simulink model "nms_3Dmodel_forward_no_rbld"  (R2017b)
settings: Solver=VariableStepAuto  StartTime=0.0  StopTime=t_end  FixedStep=1e-4  MinStep=1e-9  RelTol=1e-2  AbsTol=1e-3  EnableMultiTasking=on
InitFcn:
  | runScripts;
values from neighbouring files (symbols this model uses):
  ankle_height = 0.08    [nms_MechInit.m]
  ankleIMP = param(91+length(paramIC_opt):93+length(paramIC_opt))    [runScripts.m]
  c = 0.05    [IID_nms_MechInit.m]    (also in nms_MechInit.m)
  c_jointstop = 0.3 / (pi/180)    (= 17.1887338539)    [IID_nms_MechInit.m]    (also in nms_MechInit.m)
  CPG_On = 0    [setCPGPar.m]    (also in setCPGPar_inv.m = 1)
  CtrlPar_FP = [alpha0 alpha_cd alpha_cv]    [setCtrlPar.m]
  CtrlPar_FP_R = [R_hipR0 R_hipR_cd R_hipR_cv]    [setCtrlPar.m]
  CtrlPar_LL = l_clr    [setCtrlPar.m]
  CtrlPar_Side = [beta_cd  beta_cv]    [setCtrlPar.m]
  CtrlPar_St = [StPreStim St_M1 St_M2 St_M3 St_M4 St_M5 St_M11]    [setCtrlPar.m]
  CtrlPar_St_R = [R_StPreStim R_St_M1 R_St_M3 R_St_M4]    [setCtrlPar.m]
  CtrlPar_Sw = [SwPreStim SwPhasePari SwPhaseParii SwCtrlPar_H SwCtrlPar_A      SwCtrlPar_Ki SwCtrlPar_Kii SwCtrlPar_Kiii SwCtrlPar_StP]    [setCtrlPar.m]
  CtrlPar_Sw_R = [R_SwPreStim R_Sw_M6]    [setCtrlPar.m]
  CtrlPar_theta0 = parBlCtrl(1)      *1*pi/180    [setCtrlPar.m]
  CtrlPar_Tr = [Tr_St_sup Tr_Sw]    [setCtrlPar.m]
  CtrlPar_Tr_R = [R_Tr_St_sup R_Tr_Sw]    [setCtrlPar.m]
  D12_F = 0.16    [IID_nms_MechInit.m]    (also in nms_MechInit.m)
  D12_S = L_S    (= 0.5)    [IID_nms_MechInit.m]    (also in nms_MechInit.m = 0.46)
  D12_T = L_T    (= 0.5)    [IID_nms_MechInit.m]    (also in nms_MechInit.m = 0.46)
  D12z_T = 0.1* scalorFactor    (= 0.1)    [nms_MechInit.m]
  D13_F = 0.20    (= 0.2)    [IID_nms_MechInit.m]    (also in nms_MechInit.m)
  D1G_F = 0.14    [IID_nms_MechInit.m]    (also in nms_MechInit.m)
  D1G_HAT = 0.35    [IID_nms_MechInit.m]    (also in nms_MechInit.m)
  D1G_S = 0.3    [IID_nms_MechInit.m]    (also in nms_MechInit.m = 0.28)
  D1G_T = 0.3    [IID_nms_MechInit.m]    (also in nms_MechInit.m = 0.28)
  D1Gy_F = ankle_height*D1G_F/D12_F    (= 0.07)    [nms_MechInit.m]
  d_fBall = 0.1    [nms_MechInit.m]
  d_fHeel = 0.05    [nms_MechInit.m]
  DeltaThRef = 5e-3    (= 0.005)    [IID_nms_MechInit.m]    (also in nms_MechInit.m)
  Dist_LM23_PH = 0    [setDistPar.m]
  Dist_LM34_PH = 0    [setDistPar.m]
  Dist_On = 1    [IID_setDistPar.m]    (also in setDistPar.m)
  Dist_PDur = 0.15    [IID_setDistPar.m]    (also in setDistPar.m)
  Dist_RM23_PH = 0    [setDistPar.m]
  Dist_RM34_PH = 0    [setDistPar.m]
  Dist_StartTime = 15    [IID_setDistPar.m]    (also in setDistPar.m)
  Dist_xyzHAT_front_PH = 0    [setDistPar.m]
  Dist_xyzHAT_sag_PH = 0    [IID_setDistPar.m]    (also in setDistPar.m)
  Dist_xyzLAnkle_PH = 0    [setDistPar.m]
  Dist_xyzRAnkle_PH = 0    [setDistPar.m]
  eref = 0.04    [IID_nms_MechInit.m]    (also in nms_MechInit.m)
  FmaxBFSH = 350    [nms_MechInit.m]
  FmaxGAS = 1500    [IID_nms_MechInit.m]    (also in nms_MechInit.m)
  FmaxGLU = 1500    [IID_nms_MechInit.m]    (also in nms_MechInit.m)
  FmaxHAB = 3000    [nms_MechInit.m]
  FmaxHAD = 4500    [nms_MechInit.m]
  FmaxHAM = 3000    [IID_nms_MechInit.m]    (also in nms_MechInit.m)
  FmaxHFL = 2000    [IID_nms_MechInit.m]    (also in nms_MechInit.m)
  FmaxRF = 1200    [nms_MechInit.m]
  FmaxSOL = 4000    [IID_nms_MechInit.m]    (also in nms_MechInit.m)
  FmaxTA = 800    [IID_nms_MechInit.m]    (also in nms_MechInit.m)
  FmaxVAS = 6000    [IID_nms_MechInit.m]    (also in nms_MechInit.m)
  In_F = 0.005    [IID_nms_MechInit.m]    (also in nms_MechInit.m)
  In_HAT = 3    [IID_nms_MechInit.m]    (also in nms_MechInit.m = 2.5)
  In_S = 0.05    [IID_nms_MechInit.m]    (also in nms_MechInit.m)
  In_T = 0.15    [IID_nms_MechInit.m]    (also in nms_MechInit.m)
  init_a_tgt = 70*pi/180    (= 1.2217304764)    [setInitPar.m]
  init_a_tgtR = 90*pi/180    (= 1.57079632679)    [setInitPar.m]
  Inx_F = 0.0007    [nms_MechInit.m]
  Inx_HAT = 1.0    (= 1)    [nms_MechInit.m]
  Inx_S = 0.003    [nms_MechInit.m]
  Inx_T = 0.03    [nms_MechInit.m]
  Iny_F = 0.005    [nms_MechInit.m]
  Iny_HAT = 4.0    (= 4)    [nms_MechInit.m]
  Iny_S = 0.05    [nms_MechInit.m]
  Iny_T = 0.15    [nms_MechInit.m]
  K = 5    [IID_nms_MechInit.m]    (also in nms_MechInit.m)
  k_gn = k_gn/2    (= 39240)    [nms_MechInit.m]
  k_gt = k_gt/2    (= 3924)    [nms_MechInit.m]
  k_pressure = m_HAT * 9.81 / DeltaThRef    (= 104967)    [IID_nms_MechInit.m]    (also in nms_MechInit.m)
  leg_l = [D12_T D12_S]    [nms_MechInit.m]
  LongDelay = 0.020    (= 0.02)    [IID_setCtrlPar.m]    (also in nms_MechInit.m = 0.01)
  LongLoopDelay = 0.030    (= 0.03)    [nms_MechInit.m]
  loptBFSH = 0.12    [nms_MechInit.m]
  loptGAS = 0.05    [IID_nms_MechInit.m]    (also in nms_MechInit.m)
  loptGLU = 0.11    [IID_nms_MechInit.m]    (also in nms_MechInit.m)
  loptHAB = 0.09    [nms_MechInit.m]
  loptHAD = 0.10    (= 0.1)    [nms_MechInit.m]
  loptHAM = 0.10    (= 0.1)    [IID_nms_MechInit.m]    (also in nms_MechInit.m)
  loptHFL = 0.11    [IID_nms_MechInit.m]    (also in nms_MechInit.m)
  loptRF = 0.08    [nms_MechInit.m]
  loptSOL = 0.04    [IID_nms_MechInit.m]    (also in nms_MechInit.m)
  loptTA = 0.06    [IID_nms_MechInit.m]    (also in nms_MechInit.m)
  loptVAS = 0.08    [IID_nms_MechInit.m]    (also in nms_MechInit.m)
  lslackBFSH = 0.10    (= 0.1)    [nms_MechInit.m]
  lslackGAS = 0.40    (= 0.4)    [IID_nms_MechInit.m]    (also in nms_MechInit.m)
  lslackGLU = 0.13    [IID_nms_MechInit.m]    (also in nms_MechInit.m)
  lslackHAB = 0.07    [nms_MechInit.m]
  lslackHAD = 0.18    [nms_MechInit.m]
  lslackHAM = 0.31    [IID_nms_MechInit.m]    (also in nms_MechInit.m)
  lslackHFL = 0.10    (= 0.1)    [IID_nms_MechInit.m]    (also in nms_MechInit.m)
  lslackRF = 0.35    [nms_MechInit.m]
  lslackSOL = 0.26    [IID_nms_MechInit.m]    (also in nms_MechInit.m)
  lslackTA = 0.24    [IID_nms_MechInit.m]    (also in nms_MechInit.m)
  lslackVAS = 0.23    [IID_nms_MechInit.m]    (also in nms_MechInit.m)
  m_F = 1.25    [IID_nms_MechInit.m]    (also in nms_MechInit.m)
  m_HAT = 53.5    [IID_nms_MechInit.m]    (also in nms_MechInit.m)
  m_S = 3.5    [IID_nms_MechInit.m]    (also in nms_MechInit.m)
  m_T = 8.5    [IID_nms_MechInit.m]    (also in nms_MechInit.m)
  m_Total = m_F*2+m_S*2+m_T*2+m_HAT    (= 80)    [IID_nms_MechInit.m]    (also in nms_MechInit.m)
  massBFSH = 2    [nms_MechInit.m]
  massGAS = 0.45    [IID_nms_MechInit.m]    (also in nms_MechInit.m)
  massGLU = 1.4    [IID_nms_MechInit.m]    (also in nms_MechInit.m)
  massHAB = 1.145    [nms_MechInit.m]
  massHAD = 1.91    [nms_MechInit.m]
  massHAM = 1.82    [IID_nms_MechInit.m]    (also in nms_MechInit.m)
  massHFL = 1.87    [IID_nms_MechInit.m]    (also in nms_MechInit.m)
  massRF = 1    [nms_MechInit.m]
  massSOL = 1.36    [IID_nms_MechInit.m]    (also in nms_MechInit.m)
  massTA = 0.29    [IID_nms_MechInit.m]    (also in nms_MechInit.m)
  massVAS = 2.91    [IID_nms_MechInit.m]    (also in nms_MechInit.m)
  MidDelay = 0.010    (= 0.01)    [IID_setCtrlPar.m]    (also in nms_MechInit.m = 0.005)
  mu_slide = 0.8    [IID_nms_MechInit.m]    (also in nms_MechInit.m)
  mu_stick = 0.9    [IID_nms_MechInit.m]    (also in nms_MechInit.m)
  N = 1.5    [IID_nms_MechInit.m]    (also in cmaes_parfor.m = size(x,1); nms_MechInit.m)
  phi12_LowLimit = 70*pi/180    (= 1.2217304764)    [IID_nms_MechInit.m]    (also in nms_MechInit.m)
  phi12_UpLimit = 130*pi/180    (= 2.26892802759)    [IID_nms_MechInit.m]    (also in nms_MechInit.m)
  phi23_UpLimit = 175*pi/180    (= 3.05432619099)    [IID_nms_MechInit.m]    (also in nms_MechInit.m)
  phi34_UpLimit = 230*pi/180    (= 4.01425727959)    [IID_nms_MechInit.m]    (also in nms_MechInit.m)
  phi34R_LowLimit = -15*pi/180    (= -0.261799387799)    [nms_MechInit.m]
  ... (+115 more)
undefined symbols (not defined in the file or in its folder): magnitude, sgn
libraries: mblibv1 x104, simulink x54, simulink_extras x38, nmc x30, NMCCPG_Library x17, powerlib_meascontrol x5
(part 7 of 17)

== system nms_3Dmodel_forward_no_rbld/Muscle Actuation Layer/L RF Link ==
  note: RF Attachment
  phi34 [rad] : Inport
  phi23 [rad] : Inport  Port=2
  Constant1 : Constant  Value=phimaxRFk
  Constant2 : Constant  Value=phirefRFk
  Constant3 : Constant  Value=rRFh
  Constant4 : Constant  Value=lslackRF+loptRF
  Constant5 : Constant  Value=phirefRFh
  Demux : Demux  Outputs=2
  Gain1 : Gain  Gain=rRFkmax
  Gain2 : Gain  Gain=rhoRFh
  Gain3 : Gain  Gain=phiScaleRFk
  Gain4 : Gain  Gain=rhoRFk/phiScaleRFk
  Gain5 : Gain  Gain=phiScaleRFk
  Mux : Mux  Inputs=2
  Product : Product  RndMeth=Zero
  Sum1 : Sum  Inputs=-+
  Sum2 : Sum  Inputs=|+-
  Sum3 : Sum  Inputs=-+|
  Sum4 : Sum  Inputs=|+-
  Sum5 : Sum  Inputs=++-
  length change term : Trigonometry
  offset correction term : Trigonometry
  variable lever term : Trigonometry  Operator=cos
  lmtu [m] : Outport
  lever34 [m] : Outport  Port=2
  lever23 [m] : Outport  Port=3
  wires:
  Sum5/1 -> lmtu [m]/1
  Constant4/1 -> Sum5/2
  Gain4/1 -> Sum5/3
  Gain2/1 -> Sum5/1
  phi34 [rad]/1 -> Sum4/1
  Constant5/1 -> Sum4/2
  Sum4/1 -> Product/1
  Constant3/1 -> Product/2, lever34 [m]/1
  Product/1 -> Gain2/1
  phi23 [rad]/1 -> Sum3/2
  Sum3/1 -> Gain3/1
  Constant1/1 -> Sum3/1, Sum2/2
  Sum2/1 -> Gain5/1
  Constant2/1 -> Sum2/1
  length change term/1 -> Sum1/2
  offset correction term/1 -> Sum1/1
  Sum1/1 -> Mux/1
  variable lever term/1 -> Mux/2
  Mux/1 -> Gain1/1
  Gain1/1 -> Demux/1
  Demux/2 -> lever23 [m]/1
  Demux/1 -> Gain4/1
  Gain3/1 -> variable lever term/1, length change term/1
  Gain5/1 -> offset correction term/1

== system nms_3Dmodel_forward_no_rbld/Muscle Actuation Layer/L SOL ==
  note: SOL Muscle-Tendon Dynamics
  note: Excitation Contraction Coupling
  STIM : Inport
  lmtc [m] : Inport  Port=2
  1 : Product  Inputs=**  SaturateOnIntegerOverflow=on  InputSameDT=on  OutDataTypeStr=Inherit: Same as first input
  1/lslack : Gain  Gain=1/lslackSOL  SaturateOnIntegerOverflow=on  OutDataTypeStr=Inherit: Same as input  ParamDataTypeStr=Inherit: Same as input
  2 : Product  Inputs=***  SaturateOnIntegerOverflow=on  InputSameDT=on  OutDataTypeStr=Inherit: Same as first input
  BE force-length relation : Subsystem
  CE force-length relation : Subsystem
  CE inverse force-velocity relation : Subsystem
  Constant : Constant  Value=lslackSOL
  ECC TransferFcn : simulink_extras/Additional Linear/Transfer Fcn (with initial outputs)  N=[1]  D="[tau  1]"  Y0=preA  U0=0
      settings: AttributesFormatString=pre-activation: %<Y0>
  Fmax : Gain  Gain=FmaxSOL  SaturateOnIntegerOverflow=on  OutDataTypeStr=Inherit: Same as input  ParamDataTypeStr=Inherit: Same as input
  Fmax1 : Gain  Gain=FmaxSOL  SaturateOnIntegerOverflow=on  OutDataTypeStr=Inherit: Same as input  ParamDataTypeStr=Inherit: Same as input
  Fv = Fse / (A*Fce) : Product  Inputs=*/  SaturateOnIntegerOverflow=on  InputSameDT=on  OutDataTypeStr=Inherit: Same as first input
  Integrator : Integrator  InitialConditionSource=external  LowerSaturationLimit=0.05  ZeroCross=off
  PE force-length relation : Subsystem
  SE force-length relation : Subsystem
  Sum : Sum  Inputs=|+-  SaturateOnIntegerOverflow=on  InputSameDT=on  OutDataTypeStr=Inherit: Same as first input
  Sum2 : Sum  Inputs=|-+  SaturateOnIntegerOverflow=on  InputSameDT=on  OutDataTypeStr=Inherit: Same as first input
  Sum3 : Sum  SaturateOnIntegerOverflow=on  InputSameDT=on  OutDataTypeStr=Inherit: Same as first input
  Sum4 : Sum  SaturateOnIntegerOverflow=on  InputSameDT=on  OutDataTypeStr=Inherit: Same as first input
  lce/lopt : Gain  Gain=1/loptSOL  SaturateOnIntegerOverflow=on  OutDataTypeStr=Inherit: Same as input  ParamDataTypeStr=Inherit: Same as input
  vmax*lopt : Gain  Gain=vmaxSOL*loptSOL  SaturateOnIntegerOverflow=on  OutDataTypeStr=Inherit: Same as input  ParamDataTypeStr=Inherit: Same as input
  Fmtc : Outport  InitialOutput=0
  Lce : Outport  Port=2  InitialOutput=0
  Vce : Outport  Port=3  InitialOutput=0
  A : Outport  Port=4  InitialOutput=0
  Fac : Outport  Port=5  InitialOutput=0
  wires:
  Integrator/1 -> Sum/2, lce/lopt/1, Lce/1  "lce"
  Sum/1 -> 1/lslack/1  "lse"
  lce/lopt/1 -> CE force-length relation/1(lce [lopt]), BE force-length relation/1(lce [lopt]), PE force-length relation/1(lce [lopt])
  vmax*lopt/1 -> Integrator/1, Vce/1  "vce"
  lmtc [m]/1 -> Sum2/2, Sum/1  "lmtc"
  Fmax/1 -> Fmtc/1  "Fmtc"
  1/lslack/1 -> SE force-length relation/1(lse [lslack])
  SE force-length relation/1(fse [Fmax]) -> Fmax/1, Sum4/1
  Sum2/1 -> Integrator/2
  Constant/1 -> Sum2/1
  Sum4/1 -> Fv = Fse / (A*Fce)/1
  PE force-length relation/1(fpe [Fmax]) -> Sum3/1
  1/1 -> Sum3/2
  BE force-length relation/1(fbe [Fmax]) -> Sum4/2
  Sum3/1 -> Fv = Fse / (A*Fce)/2
  CE inverse force-velocity relation/1(v[vmax]) -> vmax*lopt/1
  STIM/1 -> ECC TransferFcn/1
  Fv = Fse / (A*Fce)/1 -> 2/3, CE inverse force-velocity relation/1(Fv[Fmax])  "fv"
  CE force-length relation/1(fce [Fmax]) -> 2/1, 1/1  "fl"
  ECC TransferFcn/1 -> 2/2, A/1, 1/2  "A"
  2/1 -> Fmax1/1
  Fmax1/1 -> Fac/1

== system nms_3Dmodel_forward_no_rbld/Muscle Actuation Layer/L SOL Link ==
  note: Soleus Attachment
  phi12 [rad] : Inport
  Constant : Constant  Value=lslackSOL+loptSOL
  Constant3 : Constant  Value=phimaxSOL
  Constant5 : Constant  Value=phirefSOL
  Demux1 : Demux  Outputs=2
  Gain2 : Gain  Gain=rSOLmax
  Gain3 : Gain  Gain=phiScaleSOL
  Gain8 : Gain  Gain=phiScaleSOL
  Gain9 : Gain  Gain=rhoSOL/phiScaleSOL
  Mux1 : Mux  Inputs=2
  Sum4 : Sum  Inputs=-+
  Sum5 : Sum  Inputs=|+-
  Sum6 : Sum  Inputs=|+-
  Sum7 : Sum  Inputs=-+|
  length change term1 : Trigonometry
  offset correction term1 : Trigonometry
  variable lever term1 : Trigonometry  Operator=cos
  lmtc [m] : Outport
  lever [m] : Outport  Port=2
  wires:
  Constant/1 -> Sum5/1
  Sum5/1 -> lmtc [m]/1
  Gain9/1 -> Sum5/2
  Demux1/1 -> Gain9/1
  Demux1/2 -> lever [m]/1
  phi12 [rad]/1 -> Sum7/2
  Sum7/1 -> Gain3/1
  Constant3/1 -> Sum7/1, Sum6/2
  Sum6/1 -> Gain8/1
  Constant5/1 -> Sum6/1
  length change term1/1 -> Sum4/2
  offset correction term1/1 -> Sum4/1
  Sum4/1 -> Mux1/1
  variable lever term1/1 -> Mux1/2
  Mux1/1 -> Gain2/1
  Gain2/1 -> Demux1/1
  Gain3/1 -> variable lever term1/1, length change term1/1
  Gain8/1 -> offset correction term1/1

== system nms_3Dmodel_forward_no_rbld/Muscle Actuation Layer/L TA ==
  note: Excitation Contraction Coupling
  note: TA Muscle-Tendon Dynamics
  STIM : Inport
  lmtc [m] : Inport  Port=2
  1 : Product  Inputs=**  SaturateOnIntegerOverflow=on  InputSameDT=on  OutDataTypeStr=Inherit: Same as first input
  1/lslack : Gain  Gain=1/lslackTA  SaturateOnIntegerOverflow=on  OutDataTypeStr=Inherit: Same as input  ParamDataTypeStr=Inherit: Same as input
  2 : Product  Inputs=***  SaturateOnIntegerOverflow=on  InputSameDT=on  OutDataTypeStr=Inherit: Same as first input
  BE force-length relation : Subsystem
  CE force-length relation : Subsystem
  CE inverse force-velocity relation : Subsystem
  Constant : Constant  Value=lslackTA
  ECC TransferFcn : simulink_extras/Additional Linear/Transfer Fcn (with initial outputs)  N=[1]  D="[tau  1]"  Y0=preA  U0=0
      settings: AttributesFormatString=pre-activation: %<Y0>
  Fmax : Gain  Gain=FmaxTA  SaturateOnIntegerOverflow=on  OutDataTypeStr=Inherit: Same as input  ParamDataTypeStr=Inherit: Same as input
  Fmax1 : Gain  Gain=FmaxTA  SaturateOnIntegerOverflow=on  OutDataTypeStr=Inherit: Same as input  ParamDataTypeStr=Inherit: Same as input
  Fv = Fse / (A*Fce) : Product  Inputs=*/  SaturateOnIntegerOverflow=on  InputSameDT=on  OutDataTypeStr=Inherit: Same as first input
  Integrator : Integrator  InitialConditionSource=external  LowerSaturationLimit=0.05  ZeroCross=off
  PE force-length relation : Subsystem
  SE force-length relation : Subsystem
  Sum : Sum  Inputs=|+-  SaturateOnIntegerOverflow=on  InputSameDT=on  OutDataTypeStr=Inherit: Same as first input
  Sum2 : Sum  Inputs=|-+  SaturateOnIntegerOverflow=on  InputSameDT=on  OutDataTypeStr=Inherit: Same as first input
  Sum3 : Sum  SaturateOnIntegerOverflow=on  InputSameDT=on  OutDataTypeStr=Inherit: Same as first input
  Sum4 : Sum  SaturateOnIntegerOverflow=on  InputSameDT=on  OutDataTypeStr=Inherit: Same as first input
  lce/lopt : Gain  Gain=1/loptTA  SaturateOnIntegerOverflow=on  OutDataTypeStr=Inherit: Same as input  ParamDataTypeStr=Inherit: Same as input
  vmax*lopt : Gain  Gain=vmaxTA*loptTA  SaturateOnIntegerOverflow=on  OutDataTypeStr=Inherit: Same as input  ParamDataTypeStr=Inherit: Same as input
  Fmtc : Outport  InitialOutput=0
  Lce : Outport  Port=2  InitialOutput=0
  Vce : Outport  Port=3  InitialOutput=0
  A : Outport  Port=4  InitialOutput=0
  Fac : Outport  Port=5  InitialOutput=0
  wires:
  CE inverse force-velocity relation/1(v[vmax]) -> vmax*lopt/1
  Sum3/1 -> Fv = Fse / (A*Fce)/2
  BE force-length relation/1(fbe [Fmax]) -> Sum4/2
  1/1 -> Sum3/2
  PE force-length relation/1(fpe [Fmax]) -> Sum3/1
  Sum4/1 -> Fv = Fse / (A*Fce)/1
  CE force-length relation/1(fce [Fmax]) -> 2/1, 1/1
  Constant/1 -> Sum2/1
  Sum2/1 -> Integrator/2
  SE force-length relation/1(fse [Fmax]) -> Sum4/1, Fmax/1
  1/lslack/1 -> SE force-length relation/1(lse [lslack])
  Fmax/1 -> Fmtc/1  "Fmtc"
  lmtc [m]/1 -> Sum/1, Sum2/2  "lmtc"
  vmax*lopt/1 -> Integrator/1, Vce/1  "vce"
  lce/lopt/1 -> BE force-length relation/1(lce [lopt]), PE force-length relation/1(lce [lopt]), CE force-length relation/1(lce [lopt])
  Sum/1 -> 1/lslack/1  "lse"
  Integrator/1 -> lce/lopt/1, Sum/2, Lce/1  "lce"
  STIM/1 -> ECC TransferFcn/1
  Fv = Fse / (A*Fce)/1 -> 2/3, CE inverse force-velocity relation/1(Fv[Fmax])  "fv"
  ECC TransferFcn/1 -> 1/2, 2/2, A/1  "A"
  2/1 -> Fmax1/1
  Fmax1/1 -> Fac/1

== system nms_3Dmodel_forward_no_rbld/Muscle Actuation Layer/L TA Link ==
  note: Muscle Length and Moment Arm
  phi12 [rad] : Inport
  Constant : Constant  Value=lslackTA+loptTA
  Constant3 : Constant  Value=phimaxTA
  Constant5 : Constant  Value=phirefTA
  Demux1 : Demux  Outputs=2
  Gain2 : Gain  Gain=rTAmax
  Gain3 : Gain  Gain=phiScaleTA
  Gain8 : Gain  Gain=phiScaleTA
  Gain9 : Gain  Gain=rhoTA/phiScaleTA
  Mux1 : Mux  Inputs=2
  Sum4 : Sum  Inputs=-+
  Sum5 : Sum  Inputs=|++
  Sum6 : Sum  Inputs=|+-
  Sum7 : Sum  Inputs=-+|
  length change term1 : Trigonometry
  offset correction term1 : Trigonometry
  variable lever term1 : Trigonometry  Operator=cos
  lmtc [m] : Outport
  lever [m] : Outport  Port=2
  wires:
  Constant/1 -> Sum5/1
  Sum5/1 -> lmtc [m]/1
  Gain9/1 -> Sum5/2
  Demux1/1 -> Gain9/1
  Demux1/2 -> lever [m]/1
  phi12 [rad]/1 -> Sum7/2
  Sum7/1 -> Gain3/1
  Constant3/1 -> Sum7/1, Sum6/2
  Sum6/1 -> Gain8/1
  Constant5/1 -> Sum6/1
  length change term1/1 -> Sum4/2
  offset correction term1/1 -> Sum4/1
  Sum4/1 -> Mux1/1
  variable lever term1/1 -> Mux1/2
  Mux1/1 -> Gain2/1
  Gain2/1 -> Demux1/1
  Gain3/1 -> variable lever term1/1, length change term1/1
  Gain8/1 -> offset correction term1/1

== system nms_3Dmodel_forward_no_rbld/Muscle Actuation Layer/L VAS ==
  note: VAS Muscle-Tendon Dynamics
  note: Excitation Contraction Coupling
  STIM : Inport
  lmtc [m] : Inport  Port=2
  1 : Product  Inputs=**  SaturateOnIntegerOverflow=on  InputSameDT=on  OutDataTypeStr=Inherit: Same as first input
  1/lslack : Gain  Gain=1/lslackVAS  SaturateOnIntegerOverflow=on  OutDataTypeStr=Inherit: Same as input  ParamDataTypeStr=Inherit: Same as input
  2 : Product  Inputs=***  SaturateOnIntegerOverflow=on  InputSameDT=on  OutDataTypeStr=Inherit: Same as first input
  BE force-length relation : Subsystem
  CE force-length relation : Subsystem
  CE inverse force-velocity relation : Subsystem
  Constant : Constant  Value=lslackVAS
  ECC TransferFcn : simulink_extras/Additional Linear/Transfer Fcn (with initial outputs)  N=[1]  D="[tau  1]"  Y0=preA  U0=0
      settings: AttributesFormatString=pre-activation: %<Y0>
  Fmax : Gain  Gain=FmaxVAS  SaturateOnIntegerOverflow=on  OutDataTypeStr=Inherit: Same as input  ParamDataTypeStr=Inherit: Same as input
  Fmax1 : Gain  Gain=FmaxVAS  SaturateOnIntegerOverflow=on  OutDataTypeStr=Inherit: Same as input  ParamDataTypeStr=Inherit: Same as input
  Fv = Fse / (A*Fce) : Product  Inputs=*/  SaturateOnIntegerOverflow=on  InputSameDT=on  OutDataTypeStr=Inherit: Same as first input
  Integrator : Integrator  InitialConditionSource=external  LowerSaturationLimit=0.05  ZeroCross=off
  PE force-length relation : Subsystem
  SE force-length relation : Subsystem
  Sum : Sum  Inputs=|+-  SaturateOnIntegerOverflow=on  InputSameDT=on  OutDataTypeStr=Inherit: Same as first input
  Sum2 : Sum  Inputs=|-+  SaturateOnIntegerOverflow=on  InputSameDT=on  OutDataTypeStr=Inherit: Same as first input
  Sum3 : Sum  SaturateOnIntegerOverflow=on  InputSameDT=on  OutDataTypeStr=Inherit: Same as first input
  Sum4 : Sum  SaturateOnIntegerOverflow=on  InputSameDT=on  OutDataTypeStr=Inherit: Same as first input
  lce/lopt : Gain  Gain=1/loptVAS  SaturateOnIntegerOverflow=on  OutDataTypeStr=Inherit: Same as input  ParamDataTypeStr=Inherit: Same as input
  vmax*lopt : Gain  Gain=vmaxVAS*loptVAS  SaturateOnIntegerOverflow=on  OutDataTypeStr=Inherit: Same as input  ParamDataTypeStr=Inherit: Same as input
  Fmtc : Outport  InitialOutput=0
  Lce : Outport  Port=2  InitialOutput=0
  Vce : Outport  Port=3  InitialOutput=0
  A : Outport  Port=4  InitialOutput=0
  Fac : Outport  Port=5  InitialOutput=0
  wires:
  Integrator/1 -> Sum/2, lce/lopt/1, Lce/1  "lce"
  Sum/1 -> 1/lslack/1  "lse"
  lce/lopt/1 -> CE force-length relation/1(lce [lopt]), BE force-length relation/1(lce [lopt]), PE force-length relation/1(lce [lopt])
  vmax*lopt/1 -> Integrator/1, Vce/1  "vce"
  lmtc [m]/1 -> Sum2/2, Sum/1  "lmtc"
  Fmax/1 -> Fmtc/1  "Fmtc"
  1/lslack/1 -> SE force-length relation/1(lse [lslack])
  SE force-length relation/1(fse [Fmax]) -> Fmax/1, Sum4/1
  Sum2/1 -> Integrator/2
  Constant/1 -> Sum2/1
  CE force-length relation/1(fce [Fmax]) -> 2/1, 1/1
  Sum4/1 -> Fv = Fse / (A*Fce)/1
  PE force-length relation/1(fpe [Fmax]) -> Sum3/1
  1/1 -> Sum3/2
  BE force-length relation/1(fbe [Fmax]) -> Sum4/2
  Sum3/1 -> Fv = Fse / (A*Fce)/2
  CE inverse force-velocity relation/1(v[vmax]) -> vmax*lopt/1
  STIM/1 -> ECC TransferFcn/1
  Fv = Fse / (A*Fce)/1 -> 2/3, CE inverse force-velocity relation/1(Fv[Fmax])  "fv"
  ECC TransferFcn/1 -> 1/2, 2/2, A/1  "fl"
  2/1 -> Fmax1/1
  Fmax1/1 -> Fac/1

== system nms_3Dmodel_forward_no_rbld/Muscle Actuation Layer/L VAS Link ==
  note: Muscle Length and Moment Arm
  phi23 [rad] : Inport
  Constant : Constant  Value=lslackVAS+loptVAS
  Constant1 : Constant  Value=phimaxVAS
  Constant2 : Constant  Value=phirefVAS
  Demux : Demux  Outputs=2
  Gain1 : Gain  Gain=rVASmax
  Gain3 : Gain  Gain=phiScaleVAS
  Gain4 : Gain  Gain=rhoVAS/phiScaleVAS
  Gain5 : Gain  Gain=phiScaleVAS
  Mux : Mux  Inputs=2
  Sum1 : Sum  Inputs=-+
  Sum2 : Sum  Inputs=|+-
  Sum3 : Sum  Inputs=-+|
  Sum5 : Sum  Inputs=|+-
  length change term : Trigonometry
  offset correction term : Trigonometry
  variable lever term : Trigonometry  Operator=cos
  lmtu [m] : Outport
  lever [m] : Outport  Port=2
  wires:
  Constant/1 -> Sum5/1
  Sum5/1 -> lmtu [m]/1
  phi23 [rad]/1 -> Sum3/2
  Sum3/1 -> Gain3/1
  Constant1/1 -> Sum3/1, Sum2/2
  Sum2/1 -> Gain5/1
  Constant2/1 -> Sum2/1
  length change term/1 -> Sum1/2
  offset correction term/1 -> Sum1/1
  Sum1/1 -> Mux/1
  variable lever term/1 -> Mux/2
  Mux/1 -> Gain1/1
  Gain1/1 -> Demux/1
  Demux/2 -> lever [m]/1
  Demux/1 -> Gain4/1
  Gain3/1 -> variable lever term/1, length change term/1
  Gain5/1 -> offset correction term/1
  Gain4/1 -> Sum5/2

== system nms_3Dmodel_forward_no_rbld/Muscle Actuation Layer/Metabolic Energy LBFSH ==
  Constant : Constant  Value=loptBFSH
  Constant1 : Constant  Value=massBFSH
  Constant2 : Constant  Value=t1fBFSH
  Metabolic Energy : nmc/Metabolic Energy
      settings: SourceProductName=Neuro Muscular Controller Library
  tag scope: LEnergyBFSH=global
  wires:
  [LActBFSH] -> Metabolic Energy/1
  [LStimBFSH] -> Metabolic Energy/2
  [LLceBFSH] -> Metabolic Energy/3
  [LVceBFSH] -> Metabolic Energy/4
  [LFmBFSH] -> Metabolic Energy/5
  [LFactBFSH] -> Metabolic Energy/6
  Constant/1 -> Metabolic Energy/7
  Constant1/1 -> Metabolic Energy/8
  Constant2/1 -> Metabolic Energy/9
  Metabolic Energy/1 -> [LEnergyBFSH]

== system nms_3Dmodel_forward_no_rbld/Muscle Actuation Layer/Metabolic Energy LGAS ==
  Constant : Constant  Value=loptGAS
  Constant1 : Constant  Value=massGAS
  Constant2 : Constant  Value=t1fGAS
  Metabolic Energy : nmc/Metabolic Energy
      settings: SourceProductName=Neuro Muscular Controller Library
  tag scope: LEnergyGAS=global
  wires:
  Metabolic Energy/1 -> [LEnergyGAS]
  Constant2/1 -> Metabolic Energy/9
  Constant1/1 -> Metabolic Energy/8
  Constant/1 -> Metabolic Energy/7
  [LFactGAS] -> Metabolic Energy/6
  [LFmGAS] -> Metabolic Energy/5
  [LVceGAS] -> Metabolic Energy/4
  [LLceGAS] -> Metabolic Energy/3
  [LStimGAS] -> Metabolic Energy/2
  [LActGAS] -> Metabolic Energy/1

== system nms_3Dmodel_forward_no_rbld/Muscle Actuation Layer/Metabolic Energy LGLU ==
  Constant : Constant  Value=loptGLU
  Constant1 : Constant  Value=massGLU
  Constant2 : Constant  Value=t1fGLU
  Metabolic Energy : nmc/Metabolic Energy
      settings: SourceProductName=Neuro Muscular Controller Library
  tag scope: LEnergyGLU=global
  wires:
  [LActGLU] -> Metabolic Energy/1
  [LStimGLU] -> Metabolic Energy/2
  [LLceGLU] -> Metabolic Energy/3
  [LVceGLU] -> Metabolic Energy/4
  [LFmGLU] -> Metabolic Energy/5
  [LFactGLU] -> Metabolic Energy/6
  Constant/1 -> Metabolic Energy/7
  Constant1/1 -> Metabolic Energy/8
  Constant2/1 -> Metabolic Energy/9
  Metabolic Energy/1 -> [LEnergyGLU]

== system nms_3Dmodel_forward_no_rbld/Muscle Actuation Layer/Metabolic Energy LHAB ==
  Constant : Constant  Value=loptHAB
  Constant1 : Constant  Value=massHAB
  Constant2 : Constant  Value=t1fHAB
  Metabolic Energy : nmc/Metabolic Energy
      settings: SourceProductName=Neuro Muscular Controller Library
  tag scope: LEnergyHAB=global
  wires:
  Metabolic Energy/1 -> [LEnergyHAB]
  Constant2/1 -> Metabolic Energy/9
  Constant1/1 -> Metabolic Energy/8
  Constant/1 -> Metabolic Energy/7
  [LFactHAB] -> Metabolic Energy/6
  [LFmHAB] -> Metabolic Energy/5
  [LVceHAB] -> Metabolic Energy/4
  [LLceHAB] -> Metabolic Energy/3
  [LStimHAB] -> Metabolic Energy/2
  [LActHAB] -> Metabolic Energy/1

== system nms_3Dmodel_forward_no_rbld/Muscle Actuation Layer/Metabolic Energy LHAD ==
  Constant : Constant  Value=loptHAD
  Constant1 : Constant  Value=massHAD
  Constant2 : Constant  Value=t1fHAD
  Metabolic Energy : nmc/Metabolic Energy
      settings: SourceProductName=Neuro Muscular Controller Library
  tag scope: LEnergyHAD=global
  wires:
  [LActHAD] -> Metabolic Energy/1
  [LStimHAD] -> Metabolic Energy/2
  [LLceHAD] -> Metabolic Energy/3
  [LVceHAD] -> Metabolic Energy/4
  [LFmHAD] -> Metabolic Energy/5
  [LFactHAD] -> Metabolic Energy/6
  Constant/1 -> Metabolic Energy/7
  Constant1/1 -> Metabolic Energy/8
  Constant2/1 -> Metabolic Energy/9
  Metabolic Energy/1 -> [LEnergyHAD]

== system nms_3Dmodel_forward_no_rbld/Muscle Actuation Layer/Metabolic Energy LHAM ==
  Constant : Constant  Value=loptHAM
  Constant1 : Constant  Value=massHAM
  Constant2 : Constant  Value=t1fHAM
  Metabolic Energy : nmc/Metabolic Energy
      settings: SourceProductName=Neuro Muscular Controller Library
  tag scope: LEnergyHAM=global
  wires:
  Metabolic Energy/1 -> [LEnergyHAM]
  Constant2/1 -> Metabolic Energy/9
  Constant1/1 -> Metabolic Energy/8
  Constant/1 -> Metabolic Energy/7
  [LFactHAM] -> Metabolic Energy/6
  [LFmHAM] -> Metabolic Energy/5
  [LVceHAM] -> Metabolic Energy/4
  [LLceHAM] -> Metabolic Energy/3
  [LStimHAM] -> Metabolic Energy/2
  [LActHAM] -> Metabolic Energy/1

== system nms_3Dmodel_forward_no_rbld/Muscle Actuation Layer/Metabolic Energy LHFL ==
  Constant : Constant  Value=loptHFL
  Constant1 : Constant  Value=massHFL
  Constant2 : Constant  Value=t1fHFL
  Metabolic Energy : nmc/Metabolic Energy
      settings: SourceProductName=Neuro Muscular Controller Library
  tag scope: LEnergyHFL=global
  wires:
  Metabolic Energy/1 -> [LEnergyHFL]
  Constant2/1 -> Metabolic Energy/9
  Constant1/1 -> Metabolic Energy/8
  Constant/1 -> Metabolic Energy/7
  [LFactHFL] -> Metabolic Energy/6
  [LFmHFL] -> Metabolic Energy/5
  [LVceHFL] -> Metabolic Energy/4
  [LLceHFL] -> Metabolic Energy/3
  [LStimHFL] -> Metabolic Energy/2
  [LActHFL] -> Metabolic Energy/1

== system nms_3Dmodel_forward_no_rbld/Muscle Actuation Layer/Metabolic Energy LRF ==
  Constant : Constant  Value=loptRF
  Constant1 : Constant  Value=massRF
  Constant2 : Constant  Value=t1fRF
  Metabolic Energy : nmc/Metabolic Energy
      settings: SourceProductName=Neuro Muscular Controller Library
  tag scope: LEnergyRF=global
  wires:
  [LActRF] -> Metabolic Energy/1
  [LStimRF] -> Metabolic Energy/2
  [LLceRF] -> Metabolic Energy/3
  [LVceRF] -> Metabolic Energy/4
  [LFmRF] -> Metabolic Energy/5
  [LFactRF] -> Metabolic Energy/6
  Constant/1 -> Metabolic Energy/7
  Constant1/1 -> Metabolic Energy/8
  Constant2/1 -> Metabolic Energy/9
  Metabolic Energy/1 -> [LEnergyRF]

== system nms_3Dmodel_forward_no_rbld/Muscle Actuation Layer/Metabolic Energy LSOL ==
  Constant : Constant  Value=loptSOL
  Constant1 : Constant  Value=massSOL
  Constant2 : Constant  Value=t1fSOL
  Metabolic Energy : nmc/Metabolic Energy
      settings: SourceProductName=Neuro Muscular Controller Library
  tag scope: LEnergySOL=global
  wires:
  [LActSOL] -> Metabolic Energy/1
  [LStimSOL] -> Metabolic Energy/2
  [LLceSOL] -> Metabolic Energy/3
  [LVceSOL] -> Metabolic Energy/4
  [LFmSOL] -> Metabolic Energy/5
  [LFactSOL] -> Metabolic Energy/6
  Constant/1 -> Metabolic Energy/7
  Constant1/1 -> Metabolic Energy/8
  Constant2/1 -> Metabolic Energy/9
  Metabolic Energy/1 -> [LEnergySOL]

== system nms_3Dmodel_forward_no_rbld/Muscle Actuation Layer/Metabolic Energy LTA ==
  Constant : Constant  Value=loptTA
  Constant1 : Constant  Value=massTA
  Constant2 : Constant  Value=t1fTA
  Metabolic Energy : nmc/Metabolic Energy
      settings: SourceProductName=Neuro Muscular Controller Library
  tag scope: LEnergyTA=global
  wires:
  [LActTA] -> Metabolic Energy/1
  [LStimTA] -> Metabolic Energy/2
  [LLceTA] -> Metabolic Energy/3
  [LVceTA] -> Metabolic Energy/4
  [LFmTA] -> Metabolic Energy/5
  [LFactTA] -> Metabolic Energy/6
  Constant/1 -> Metabolic Energy/7
  Constant1/1 -> Metabolic Energy/8
  Constant2/1 -> Metabolic Energy/9
  Metabolic Energy/1 -> [LEnergyTA]

== system nms_3Dmodel_forward_no_rbld/Muscle Actuation Layer/Metabolic Energy LVAS ==
  Constant : Constant  Value=loptVAS
  Constant1 : Constant  Value=massVAS
  Constant2 : Constant  Value=t1fVAS
  Metabolic Energy : nmc/Metabolic Energy
      settings: SourceProductName=Neuro Muscular Controller Library
  tag scope: LEnergyVAS=global
  wires:
  Metabolic Energy/1 -> [LEnergyVAS]
  Constant2/1 -> Metabolic Energy/9
  Constant1/1 -> Metabolic Energy/8
  Constant/1 -> Metabolic Energy/7
  [LFactVAS] -> Metabolic Energy/6
  [LFmVAS] -> Metabolic Energy/5
  [LVceVAS] -> Metabolic Energy/4
  [LLceVAS] -> Metabolic Energy/3
  [LStimVAS] -> Metabolic Energy/2
  [LActVAS] -> Metabolic Energy/1

== system nms_3Dmodel_forward_no_rbld/Muscle Actuation Layer/Metabolic Energy RBFSH ==
  Constant : Constant  Value=loptBFSH
  Constant1 : Constant  Value=massBFSH
  Constant2 : Constant  Value=t1fBFSH
  Metabolic Energy : nmc/Metabolic Energy
      settings: SourceProductName=Neuro Muscular Controller Library
  tag scope: REnergyBFSH=global
  wires:
  [RActBFSH] -> Metabolic Energy/1
  [RStimBFSH] -> Metabolic Energy/2
  [RLceBFSH] -> Metabolic Energy/3
  [RVceBFSH] -> Metabolic Energy/4
  [RFmBFSH] -> Metabolic Energy/5
  [RFactBFSH] -> Metabolic Energy/6
  Constant/1 -> Metabolic Energy/7
  Constant1/1 -> Metabolic Energy/8
  Constant2/1 -> Metabolic Energy/9
  Metabolic Energy/1 -> [REnergyBFSH]

== system nms_3Dmodel_forward_no_rbld/Muscle Actuation Layer/Metabolic Energy RGAS ==
  Constant : Constant  Value=loptGAS
  Constant1 : Constant  Value=massGAS
  Constant2 : Constant  Value=t1fGAS
  Metabolic Energy : nmc/Metabolic Energy
      settings: SourceProductName=Neuro Muscular Controller Library
  tag scope: REnergyGAS=global
  wires:
  Metabolic Energy/1 -> [REnergyGAS]
  Constant2/1 -> Metabolic Energy/9
  Constant1/1 -> Metabolic Energy/8
  Constant/1 -> Metabolic Energy/7
  [RFactGAS] -> Metabolic Energy/6
  [RFmGAS] -> Metabolic Energy/5
  [RVceGAS] -> Metabolic Energy/4
  [RLceGAS] -> Metabolic Energy/3
  [RStimGAS] -> Metabolic Energy/2
  [RActGAS] -> Metabolic Energy/1

== system nms_3Dmodel_forward_no_rbld/Muscle Actuation Layer/Metabolic Energy RGLU ==
  Constant : Constant  Value=loptGLU
  Constant1 : Constant  Value=massGLU
  Constant2 : Constant  Value=t1fGLU
  Metabolic Energy : nmc/Metabolic Energy
      settings: SourceProductName=Neuro Muscular Controller Library
  tag scope: REnergyGLU=global
  wires:
  [RActGLU] -> Metabolic Energy/1
  [RStimGLU] -> Metabolic Energy/2
  [RLceGLU] -> Metabolic Energy/3
  [RVceGLU] -> Metabolic Energy/4
  [RFmGLU] -> Metabolic Energy/5
  [RFactGLU] -> Metabolic Energy/6
  Constant/1 -> Metabolic Energy/7
  Constant1/1 -> Metabolic Energy/8
  Constant2/1 -> Metabolic Energy/9
  Metabolic Energy/1 -> [REnergyGLU]

== system nms_3Dmodel_forward_no_rbld/Muscle Actuation Layer/Metabolic Energy RHAB ==
  Constant : Constant  Value=loptHAB
  Constant1 : Constant  Value=massHAB
  Constant2 : Constant  Value=t1fHAB
  Metabolic Energy : nmc/Metabolic Energy
      settings: SourceProductName=Neuro Muscular Controller Library
  tag scope: REnergyHAB=global
  wires:
  Metabolic Energy/1 -> [REnergyHAB]
  Constant2/1 -> Metabolic Energy/9
  Constant1/1 -> Metabolic Energy/8
  Constant/1 -> Metabolic Energy/7
  [RFactHAB] -> Metabolic Energy/6
  [RFmHAB] -> Metabolic Energy/5
  [RVceHAB] -> Metabolic Energy/4
  [RLceHAB] -> Metabolic Energy/3
  [RStimHAB] -> Metabolic Energy/2
  [RActHAB] -> Metabolic Energy/1

== system nms_3Dmodel_forward_no_rbld/Muscle Actuation Layer/Metabolic Energy RHAB1 ==
  Constant : Constant  Value=loptHAD
  Constant1 : Constant  Value=massHAD
  Constant2 : Constant  Value=t1fHAD
  Metabolic Energy : nmc/Metabolic Energy
      settings: SourceProductName=Neuro Muscular Controller Library
  tag scope: REnergyHAD=global
  wires:
  [RActHAD] -> Metabolic Energy/1
  [RStimHAD] -> Metabolic Energy/2
  [RLceHAD] -> Metabolic Energy/3
  [RVceHAD] -> Metabolic Energy/4
  [RFmHAD] -> Metabolic Energy/5
  [RFactHAD] -> Metabolic Energy/6
  Constant/1 -> Metabolic Energy/7
  Constant1/1 -> Metabolic Energy/8
  Constant2/1 -> Metabolic Energy/9
  Metabolic Energy/1 -> [REnergyHAD]

== system nms_3Dmodel_forward_no_rbld/Muscle Actuation Layer/Metabolic Energy RHAM ==
  Constant : Constant  Value=loptHAM
  Constant1 : Constant  Value=massHAM
  Constant2 : Constant  Value=t1fHAM
  Metabolic Energy : nmc/Metabolic Energy
      settings: SourceProductName=Neuro Muscular Controller Library
  tag scope: REnergyHAM=global
  wires:
  Metabolic Energy/1 -> [REnergyHAM]
  Constant2/1 -> Metabolic Energy/9
  Constant1/1 -> Metabolic Energy/8
  Constant/1 -> Metabolic Energy/7
  [RFactHAM] -> Metabolic Energy/6
  [RFmHAM] -> Metabolic Energy/5
  [RVceHAM] -> Metabolic Energy/4
  [RLceHAM] -> Metabolic Energy/3
  [RStimHAM] -> Metabolic Energy/2
  [RActHAM] -> Metabolic Energy/1

== system nms_3Dmodel_forward_no_rbld/Muscle Actuation Layer/Metabolic Energy RHFL ==
  Constant : Constant  Value=loptHFL
  Constant1 : Constant  Value=massHFL
  Constant2 : Constant  Value=t1fHFL
  Metabolic Energy : nmc/Metabolic Energy
      settings: SourceProductName=Neuro Muscular Controller Library
  tag scope: REnergyHFL=global
  wires:
  Metabolic Energy/1 -> [REnergyHFL]
  Constant2/1 -> Metabolic Energy/9
  Constant1/1 -> Metabolic Energy/8
  Constant/1 -> Metabolic Energy/7
  [RFactHFL] -> Metabolic Energy/6
  [RFmHFL] -> Metabolic Energy/5
  [RVceHFL] -> Metabolic Energy/4
  [RLceHFL] -> Metabolic Energy/3
  [RStimHFL] -> Metabolic Energy/2
  [RActHFL] -> Metabolic Energy/1

== system nms_3Dmodel_forward_no_rbld/Muscle Actuation Layer/Metabolic Energy RRF ==
  Constant : Constant  Value=loptRF
  Constant1 : Constant  Value=massRF
  Constant2 : Constant  Value=t1fRF
  Metabolic Energy : nmc/Metabolic Energy
      settings: SourceProductName=Neuro Muscular Controller Library
  tag scope: REnergyRF=global
  wires:
  [RActRF] -> Metabolic Energy/1
  [RStimRF] -> Metabolic Energy/2
  [RLceRF] -> Metabolic Energy/3
  [RVceRF] -> Metabolic Energy/4
  [RFmRF] -> Metabolic Energy/5
  [RFactRF] -> Metabolic Energy/6
  Constant/1 -> Metabolic Energy/7
  Constant1/1 -> Metabolic Energy/8
  Constant2/1 -> Metabolic Energy/9
  Metabolic Energy/1 -> [REnergyRF]

== system nms_3Dmodel_forward_no_rbld/Muscle Actuation Layer/Metabolic Energy RSOL ==
  Constant : Constant  Value=loptSOL
  Constant1 : Constant  Value=massSOL
  Constant2 : Constant  Value=t1fSOL
  Metabolic Energy : nmc/Metabolic Energy
      settings: SourceProductName=Neuro Muscular Controller Library
  tag scope: REnergySOL=global
  wires:
  [RActSOL] -> Metabolic Energy/1
  [RStimSOL] -> Metabolic Energy/2
  [RLceSOL] -> Metabolic Energy/3
  [RVceSOL] -> Metabolic Energy/4
  [RFmSOL] -> Metabolic Energy/5
  [RFactSOL] -> Metabolic Energy/6
  Constant/1 -> Metabolic Energy/7
  Constant1/1 -> Metabolic Energy/8
  Constant2/1 -> Metabolic Energy/9
  Metabolic Energy/1 -> [REnergySOL]

== system nms_3Dmodel_forward_no_rbld/Muscle Actuation Layer/Metabolic Energy RTA ==
  Constant : Constant  Value=loptTA
  Constant1 : Constant  Value=massTA
  Constant2 : Constant  Value=t1fTA
  Metabolic Energy : nmc/Metabolic Energy
      settings: SourceProductName=Neuro Muscular Controller Library
  tag scope: REnergyTA=global
  wires:
  [RActTA] -> Metabolic Energy/1
  [RStimTA] -> Metabolic Energy/2
  [RLceTA] -> Metabolic Energy/3
  [RVceTA] -> Metabolic Energy/4
  [RFmTA] -> Metabolic Energy/5
  [RFactTA] -> Metabolic Energy/6
  Constant/1 -> Metabolic Energy/7
  Constant1/1 -> Metabolic Energy/8
  Constant2/1 -> Metabolic Energy/9
  Metabolic Energy/1 -> [REnergyTA]

== system nms_3Dmodel_forward_no_rbld/Muscle Actuation Layer/Metabolic Energy RVAS ==
  Constant : Constant  Value=loptVAS
  Constant1 : Constant  Value=massVAS
  Constant2 : Constant  Value=t1fVAS
  Metabolic Energy : nmc/Metabolic Energy
      settings: SourceProductName=Neuro Muscular Controller Library
  tag scope: REnergyVAS=global
  wires:
  Metabolic Energy/1 -> [REnergyVAS]
  Constant2/1 -> Metabolic Energy/9
  Constant1/1 -> Metabolic Energy/8
  Constant/1 -> Metabolic Energy/7
  [RFactVAS] -> Metabolic Energy/6
  [RFmVAS] -> Metabolic Energy/5
  [RVceVAS] -> Metabolic Energy/4
  [RLceVAS] -> Metabolic Energy/3
  [RStimVAS] -> Metabolic Energy/2
  [RActVAS] -> Metabolic Energy/1

== system nms_3Dmodel_forward_no_rbld/Muscle Actuation Layer/R Ankle Joint Limits ==
  note: Ankle Joint Limits
  phi [rad] : Inport
  dphi [rad/s] : Inport  Port=2
  Gain1 : Gain  Gain=c_jointstop
  Gain2 : Gain  Gain=-1
  Gain3 : Gain  Gain=c_jointstop
  Gain4 : Gain  Gain=1/w_max_jointstop
  Limit Ankle Range : simulink/Logic and Bit Operations/Interval Test  IntervalClosedRight=on  uplimit=phi12_UpLimit + 40*pi/180  IntervalClosedLeft=on  lowlimit=phi12_LowLimit - 40*pi/180  OutDataTypeStr=boolean
  Logical Operator3 : Logic  Operator=NOT  AllPortsSameDT=off  OutDataTypeStr=boolean
  Mux1 : Mux  Inputs=2
  Mux3 : Mux  Inputs=2
  Overextension Torque : Fcn  Expr="- u(1)  *  (1-u(2)) * (u(2)<1) * (u(1)>0)"
  Overflexion Torque : Fcn  Expr="- u(1)  *  (1-u(2)) * (u(2)<1) * (u(1)<0)"
  Stop Simulation1 : Stop
  Sum : Sum  Inputs=|+-
  Sum1 : Sum  Inputs=|+-
  Sum2 : Sum
  overextension angle : Constant  Value=phi12_UpLimit
  overflexion angle : Constant  Value=phi12_LowLimit
  M_stop [Nm] : Outport
  wires:
  Mux3/1 -> Overextension Torque/1
  Gain3/1 -> Mux3/1
  dphi [rad/s]/1 -> Gain4/1
  overextension angle/1 -> Sum/2
  phi [rad]/1 -> Sum/1, Sum1/1, Limit Ankle Range/1
  Sum/1 -> Gain3/1
  Gain4/1 -> Gain2/1, Mux1/2
  Gain1/1 -> Mux1/1
  Sum1/1 -> Gain1/1
  overflexion angle/1 -> Sum1/2
  Mux1/1 -> Overflexion Torque/1
  Sum2/1 -> M_stop [Nm]/1
  Gain2/1 -> Mux3/2
  Overflexion Torque/1 -> Sum2/2
  Overextension Torque/1 -> Sum2/1
  Limit Ankle Range/1 -> Logical Operator3/1
  Logical Operator3/1 -> Stop Simulation1/1

== system nms_3Dmodel_forward_no_rbld/Muscle Actuation Layer/R BFSH ==
  note: BFSH Muscle-Tendon Dynamics
  note: Excitation Contraction Coupling
  STIM : Inport
  lmtc [m] : Inport  Port=2
  1 : Product  Inputs=**  SaturateOnIntegerOverflow=on  InputSameDT=on  OutDataTypeStr=Inherit: Same as first input
  1/lslack : Gain  Gain=1/lslackBFSH  SaturateOnIntegerOverflow=on  OutDataTypeStr=Inherit: Same as input  ParamDataTypeStr=Inherit: Same as input
  2 : Product  Inputs=***  SaturateOnIntegerOverflow=on  InputSameDT=on  OutDataTypeStr=Inherit: Same as first input
  BE force-length relation : Subsystem
  CE force-length relation : Subsystem
  CE inverse force-velocity relation : Subsystem
  Constant : Constant  Value=lslackBFSH
  ECC TransferFcn : simulink_extras/Additional Linear/Transfer Fcn (with initial outputs)  N=[1]  D="[tau  1]"  Y0=preA  U0=0
      settings: AttributesFormatString=pre-activation: %<Y0>
  Fmax : Gain  Gain=FmaxBFSH  SaturateOnIntegerOverflow=on  OutDataTypeStr=Inherit: Same as input  ParamDataTypeStr=Inherit: Same as input
  Fmax1 : Gain  Gain=FmaxBFSH  SaturateOnIntegerOverflow=on  OutDataTypeStr=Inherit: Same as input  ParamDataTypeStr=Inherit: Same as input
  Fv = Fse / (A*Fce) : Product  Inputs=*/  SaturateOnIntegerOverflow=on  InputSameDT=on  OutDataTypeStr=Inherit: Same as first input
  Integrator : Integrator  InitialConditionSource=external  LowerSaturationLimit=0.05  ZeroCross=off
  PE force-length relation : Subsystem
  SE force-length relation : Subsystem
  Sum : Sum  Inputs=|+-  SaturateOnIntegerOverflow=on  InputSameDT=on  OutDataTypeStr=Inherit: Same as first input
  Sum2 : Sum  Inputs=|-+  SaturateOnIntegerOverflow=on  InputSameDT=on  OutDataTypeStr=Inherit: Same as first input
  Sum3 : Sum  SaturateOnIntegerOverflow=on  InputSameDT=on  OutDataTypeStr=Inherit: Same as first input
  Sum4 : Sum  SaturateOnIntegerOverflow=on  InputSameDT=on  OutDataTypeStr=Inherit: Same as first input
  lce/lopt : Gain  Gain=1/loptBFSH  SaturateOnIntegerOverflow=on  OutDataTypeStr=Inherit: Same as input  ParamDataTypeStr=Inherit: Same as input
  vmax*lopt : Gain  Gain=vmaxBFSH*loptBFSH  SaturateOnIntegerOverflow=on  OutDataTypeStr=Inherit: Same as input  ParamDataTypeStr=Inherit: Same as input
  Fmtc : Outport  InitialOutput=0
  Lce : Outport  Port=2  InitialOutput=0
  Vce : Outport  Port=3  InitialOutput=0
  A : Outport  Port=4  InitialOutput=0
  Fac : Outport  Port=5  InitialOutput=0
  wires:
  Integrator/1 -> Sum/2, lce/lopt/1, Lce/1  "lce"
  Sum/1 -> 1/lslack/1  "lse"
  lce/lopt/1 -> CE force-length relation/1(lce [lopt]), BE force-length relation/1(lce [lopt]), PE force-length relation/1(lce [lopt])
  vmax*lopt/1 -> Integrator/1, Vce/1  "vce"
  lmtc [m]/1 -> Sum2/2, Sum/1  "lmtc"
  Fmax/1 -> Fmtc/1  "Fmtc"
  1/lslack/1 -> SE force-length relation/1(lse [lslack])
  SE force-length relation/1(fse [Fmax]) -> Fmax/1, Sum4/1
  Sum2/1 -> Integrator/2
  Constant/1 -> Sum2/1
  Sum4/1 -> Fv = Fse / (A*Fce)/1
  PE force-length relation/1(fpe [Fmax]) -> Sum3/1
  1/1 -> Sum3/2
  BE force-length relation/1(fbe [Fmax]) -> Sum4/2
  Sum3/1 -> Fv = Fse / (A*Fce)/2
  CE inverse force-velocity relation/1(v[vmax]) -> vmax*lopt/1
  STIM/1 -> ECC TransferFcn/1
  Fv = Fse / (A*Fce)/1 -> 2/3, CE inverse force-velocity relation/1(Fv[Fmax])  "fv"
  CE force-length relation/1(fce [Fmax]) -> 2/1, 1/1  "fl"
  ECC TransferFcn/1 -> 2/2, A/1, 1/2  "A"
  2/1 -> Fmax1/1
  Fmax1/1 -> Fac/1

== system nms_3Dmodel_forward_no_rbld/Muscle Actuation Layer/R BFSH Link ==
  note: BFSH Attachment
  phi23 [rad] : Inport
  Constant : Constant  Value=lslackBFSH+loptBFSH
  Constant1 : Constant  Value=rBFSH
  Constant2 : Constant  Value=phirefBFSH
  Gain4 : Gain  Gain=rhoBFSH
  Product : Product  RndMeth=Zero
  Sum2 : Sum  Inputs=|+-
  Sum5 : Sum  Inputs=|++
  lmtu [m] : Outport
  lever [m] : Outport  Port=2
  wires:
  Constant/1 -> Sum5/1
  Sum5/1 -> lmtu [m]/1
  Gain4/1 -> Sum5/2
  Product/1 -> Gain4/1
  phi23 [rad]/1 -> Sum2/1
  Constant2/1 -> Sum2/2
  Sum2/1 -> Product/1
  Constant1/1 -> Product/2, lever [m]/1

== system nms_3Dmodel_forward_no_rbld/Muscle Actuation Layer/R GAS ==
  note: GAS Muscle-Tendon Dynamics
  note: Excitation Contraction Coupling
  STIM : Inport
  lmtc [m] : Inport  Port=2
  1 : Product  Inputs=**  SaturateOnIntegerOverflow=on  InputSameDT=on  OutDataTypeStr=Inherit: Same as first input
  1/lslack : Gain  Gain=1/lslackGAS  SaturateOnIntegerOverflow=on  OutDataTypeStr=Inherit: Same as input  ParamDataTypeStr=Inherit: Same as input
  2 : Product  Inputs=***  SaturateOnIntegerOverflow=on  InputSameDT=on  OutDataTypeStr=Inherit: Same as first input
  BE force-length relation : Subsystem
  CE force-length relation : Subsystem
  CE inverse force-velocity relation : Subsystem
  Constant : Constant  Value=lslackGAS
  ECC TransferFcn : simulink_extras/Additional Linear/Transfer Fcn (with initial outputs)  N=[1]  D="[tau  1]"  Y0=preA  U0=0
      settings: AttributesFormatString=pre-activation: %<Y0>
  Fmax : Gain  Gain=FmaxGAS  SaturateOnIntegerOverflow=on  OutDataTypeStr=Inherit: Same as input  ParamDataTypeStr=Inherit: Same as input
  Fmax1 : Gain  Gain=FmaxGAS  SaturateOnIntegerOverflow=on  OutDataTypeStr=Inherit: Same as input  ParamDataTypeStr=Inherit: Same as input
  Fv = Fse / (A*Fce) : Product  Inputs=*/  SaturateOnIntegerOverflow=on  InputSameDT=on  OutDataTypeStr=Inherit: Same as first input
  Integrator : Integrator  InitialConditionSource=external  LowerSaturationLimit=0.05  ZeroCross=off
  PE force-length relation : Subsystem
  SE force-length relation : Subsystem
  Sum : Sum  Inputs=|+-  SaturateOnIntegerOverflow=on  InputSameDT=on  OutDataTypeStr=Inherit: Same as first input
  Sum2 : Sum  Inputs=|-+  SaturateOnIntegerOverflow=on  InputSameDT=on  OutDataTypeStr=Inherit: Same as first input
  Sum3 : Sum  SaturateOnIntegerOverflow=on  InputSameDT=on  OutDataTypeStr=Inherit: Same as first input
  Sum4 : Sum  SaturateOnIntegerOverflow=on  InputSameDT=on  OutDataTypeStr=Inherit: Same as first input
  lce/lopt : Gain  Gain=1/loptGAS  SaturateOnIntegerOverflow=on  OutDataTypeStr=Inherit: Same as input  ParamDataTypeStr=Inherit: Same as input
  vmax*lopt : Gain  Gain=vmaxGAS*loptGAS  SaturateOnIntegerOverflow=on  OutDataTypeStr=Inherit: Same as input  ParamDataTypeStr=Inherit: Same as input
  Fmtc : Outport  InitialOutput=0
  Lce : Outport  Port=2  InitialOutput=0
  Vce : Outport  Port=3  InitialOutput=0
  A : Outport  Port=4  InitialOutput=0
  Fac : Outport  Port=5  InitialOutput=0
  wires:
  Integrator/1 -> Sum/2, lce/lopt/1, Lce/1  "lce"
  Sum/1 -> 1/lslack/1  "lse"
  lce/lopt/1 -> CE force-length relation/1(lce [lopt]), BE force-length relation/1(lce [lopt]), PE force-length relation/1(lce [lopt])
  vmax*lopt/1 -> Integrator/1, Vce/1  "vce"
  lmtc [m]/1 -> Sum2/2, Sum/1  "lmtc"
  Fmax/1 -> Fmtc/1  "Fmtc"
  1/lslack/1 -> SE force-length relation/1(lse [lslack])
  SE force-length relation/1(fse [Fmax]) -> Fmax/1, Sum4/1
  Sum2/1 -> Integrator/2
  Constant/1 -> Sum2/1
  Sum4/1 -> Fv = Fse / (A*Fce)/1
  PE force-length relation/1(fpe [Fmax]) -> Sum3/1
  1/1 -> Sum3/2
  BE force-length relation/1(fbe [Fmax]) -> Sum4/2
  Sum3/1 -> Fv = Fse / (A*Fce)/2
  CE inverse force-velocity relation/1(v[vmax]) -> vmax*lopt/1
  STIM/1 -> ECC TransferFcn/1
  Fv = Fse / (A*Fce)/1 -> 2/3, CE inverse force-velocity relation/1(Fv[Fmax])  "fv"
  CE force-length relation/1(fce [Fmax]) -> 2/1, 1/1  "fl"
  ECC TransferFcn/1 -> 2/2, A/1, 1/2  "A"
  2/1 -> Fmax1/1
  Fmax1/1 -> Fac/1
